simulink library "testLibrary"  (R2023b)
settings: Solver=VariableStepAuto  StartTime=0.0  StopTime=10.0  RelTol=1e-3
settings Model: Creator=uditpant  LastModifiedBy=uditpant
settings DebuggingCC: UnconnectedInputMsg=warning  UnconnectedOutputMsg=warning  UnconnectedLineMsg=warning
settings ModelReferenceCC: EnableRefExpFcnMdlSchedulingChecks=on
settings RTWCC: DLArmComputeVersion=19.05

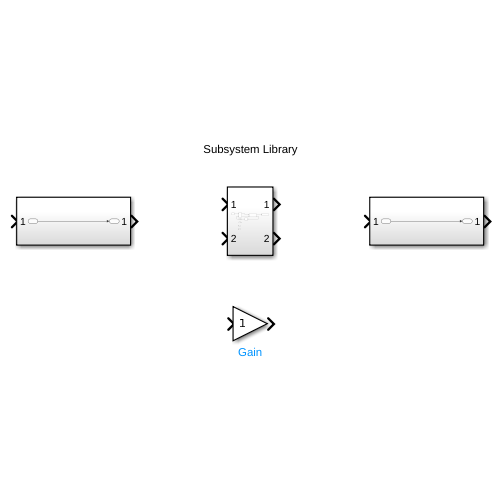
[thumbnail: Simulink's stored preview of the top-level diagram]
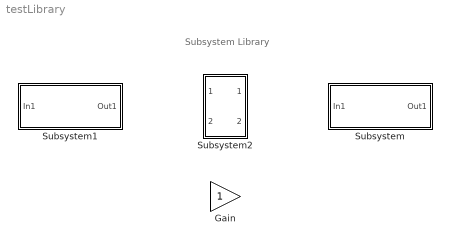
== system testLibrary ==
  note: Subsystem Library
  Gain : Gain
  Subsystem : Subsystem
  Subsystem1 : Subsystem
  Subsystem2 : Subsystem

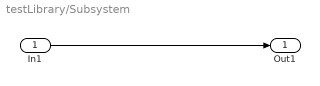
== system testLibrary/Subsystem ==
  In1 : Inport
  Out1 : Outport
  wires:
  In1/1 -> Out1/1

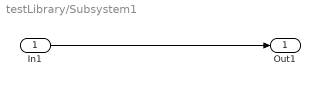
== system testLibrary/Subsystem1 ==
  In1 : Inport
  Out1 : Outport
  wires:
  In1/1 -> Out1/1

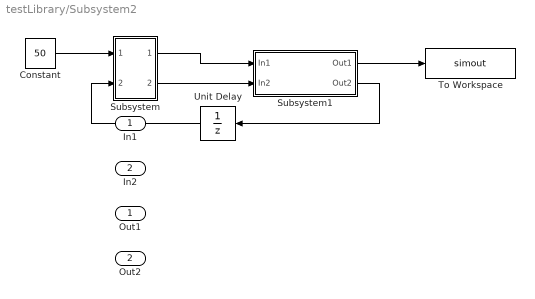
== system testLibrary/Subsystem2 ==
  In1 : Inport
  In2 : Inport  Port=2
  Constant : Constant  Value=50
  Subsystem : Subsystem
  Subsystem1 : Subsystem
  To Workspace : ToWorkspace  VariableName=simout  SaveFormat=Timeseries  SampleTime=-1
  Unit Delay : UnitDelay  SampleTime=-1  HasFrameUpgradeWarning=on
  Out1 : Outport
  Out2 : Outport  Port=2
  wires:
  Unit Delay/1 -> Subsystem/2(In2)
  Subsystem/1(Out1) -> Subsystem1/1(In1)
  Subsystem1/2(Out2) -> Unit Delay/1
  Constant/1 -> Subsystem/1(In1)
  Subsystem1/1(Out1) -> To Workspace/1
  Subsystem/2(Out2) -> Subsystem1/2(In2)

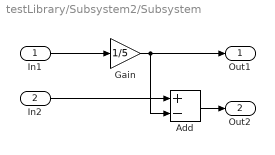
== system testLibrary/Subsystem2/Subsystem ==
  In1 : Inport
  In2 : Inport  Port=2
  Add : Sum  Inputs=+-
  Gain : Gain  Gain=1/5
  Out1 : Outport
  Out2 : Outport  Port=2
  wires:
  Gain/1 -> Add/2, Out1/1
  In1/1 -> Gain/1
  In2/1 -> Add/1
  Add/1 -> Out2/1

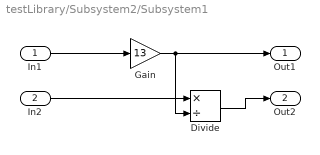
== system testLibrary/Subsystem2/Subsystem1 ==
  In1 : Inport
  In2 : Inport  Port=2
  Divide : Product  Inputs=*/
  Gain : Gain  Gain=13
  Out1 : Outport
  Out2 : Outport  Port=2
  wires:
  In1/1 -> Gain/1
  Gain/1 -> Divide/2, Out1/1
  In2/1 -> Divide/1
  Divide/1 -> Out2/1
